simulink model "ADCS_Outline"  (R2019a)
settings: Solver=VariableStepAuto  StartTime=0.0  StopTime=duration  MaxStep=step
InitFcn:
  | SC_ODIN_INITIALIZATION
values from neighbouring files (symbols this model uses):
  A = [ v(1) v(4) v(5) v(7);        v(4) v(2) v(6) v(8);        v(5) v(6) v(3) v(9);        v(7) v(8) v(9) v(10) ]    [MagnetometerCalibration.m]    (also in SC_ODIN_INITIALIZATION.m = 0.06; test.m = asin(sin(N)/sin(n)*sin(a)))
  Amag = [0.910186583854  -0.00959593267728  0.00343590491018; -0.00959593267728  1.05471221352  0.0559849466324; 0.00343590491018  0.0559849466324  1.05528532305]    [MagnetometerBias.mat]    (also in MagnetometerCalibration.m = evecs/scale*evecs')
  argentina = [1612.36;-4182.16;-4522.83]    [SC_ODIN_INITIALIZATION.m]
  As = 0.2*0.3    (= 0.06)    [SC_ODIN_INITIALIZATION.m]
  b_mag = block.InputPort(3).Data    [MagnetometerCalibration.m]    (also in SC_ODIN_INITIALIZATION.m = [10;-15.5;-12.2]*1e-6)
  bmag = [1.00003671399e-05 -1.55007781395e-05 -1.22009762149e-05]    [MagnetometerBias.mat]    (also in MagnetometerCalibration.m = centerE)
  breakpoints = data(:,1)    [SC_ODIN_INITIALIZATION.m]
  c = 2.99792458e8    (= 299792458)    [SC_ODIN_INITIALIZATION.m]
  C_I = [0.045 0.0009 -0.00007;        0.0009 0.045 -0.00003;        -0.00007 -0.00003 0.009]    [SC_ODIN_INITIALIZATION.m]
  Cd = 2.0    (= 2)    [SC_ODIN_INITIALIZATION.m]
  controller_sample_rate = 0.5    [SC_ODIN_INITIALIZATION.m]
  D = [ 2 * x,            2 * y,            2 * z,            1 + 0 * x ]    [MagnetometerCalibration.m]    (also in SC_ODIN_INITIALIZATION.m = 0.01*[1;1;1])
  datapx = data(:,2)    [SC_ODIN_INITIALIZATION.m]
  datapy = data(:,3)    [SC_ODIN_INITIALIZATION.m]
  datapz = data(:,4)    [SC_ODIN_INITIALIZATION.m]
  datavx = data(:,5)    [SC_ODIN_INITIALIZATION.m]
  datavy = data(:,6)    [SC_ODIN_INITIALIZATION.m]
  datavz = data(:,7)    [SC_ODIN_INITIALIZATION.m]
  DCM_BT0 = eye(3)    [SC_ODIN_INITIALIZATION.m]
  G = 6.67408e-11    [SC_ODIN_INITIALIZATION.m]
  ground = [1266.06;-4295.81;4526.14]    [SC_ODIN_INITIALIZATION.m]
  I = [Ixx -Ixy -Ixz;      -Ixy Iyy -Iyz;      -Ixz -Iyz Izz]    [SC_ODIN_INITIALIZATION.m]
  invA_mag = block.InputPort(2).Data    [MagnetometerCalibration.m]    (also in SC_ODIN_INITIALIZATION.m = inv(Ellrot/scale*Ellrot'))
  JD_0 = start_day+start_fraction    [SC_ODIN_INITIALIZATION.m]
  Ks = 1367    [SC_ODIN_INITIALIZATION.m]
  L = [0.0000812 -0.0022136 -0.0225868]    [SC_ODIN_INITIALIZATION.m]
  Ls = 0.01*[-3; 3; 5]    [SC_ODIN_INITIALIZATION.m]
  M = 5.9722e24    (= 5.9722e+24)    [SC_ODIN_INITIALIZATION.m]    (also in visualisation.m = uicontrol('Style','text','String',{''},'Position',[710 100+2)
  magnetorquer_tau = 0.02    [SC_ODIN_INITIALIZATION.m]
  magnetorquer_x_saturation = 0.24    [SC_ODIN_INITIALIZATION.m]
  magnetorquer_y_saturation = 0.24    [SC_ODIN_INITIALIZATION.m]
  magnetorquer_z_saturation = 0.13    [SC_ODIN_INITIALIZATION.m]
  namibia = [5659.26;1238.85;-2659.2]    [SC_ODIN_INITIALIZATION.m]
  q = 0.6    [SC_ODIN_INITIALIZATION.m]
  radii = radii .* sgns    [MagnetometerCalibration.m]    (also in SC_ODIN_INITIALIZATION.m = [1;0.9;1.1])
  W0 = [1;0;1-1/240].*pi()/180    [SC_ODIN_INITIALIZATION.m]
  wheel_saturation = 0.23e-3    (= 0.00023)    [SC_ODIN_INITIALIZATION.m]
  wheel_tau = 2    [SC_ODIN_INITIALIZATION.m]
undefined symbols (not defined in the file or in its folder): DiscIntNeverNeededParam, nut80, sun_sensors
libraries: dspmathops x94, vrlib x70, dspsrcs4 x21, realtime_pacer_lib x1, dspsolvers x1, dspinverses x1
(part 3 of 6)

== system ADCS_Outline/Guidance&Determination/Body-Earth Estimation/TRIAD DCM ==
  (Sx,Sy,Sz) : Inport
  " (Bx,By,Bz)" : Inport  Port=2
  (Sxe,Sye,Sze) : Inport  Port=3
  (Bxe,Bye,Bze) : Inport  Port=4
  Cross Product{,1..3} (4 alike) : vrlib/Utilities/Cross Product
      settings: SourceProductBaseCode=VR
  Matrix Concatenate : Concatenate  NumInputs=3  Mode=Multidimensional array  ConcatenateDimension=2
  Matrix Concatenate1 : Concatenate  NumInputs=3  Mode=Multidimensional array  ConcatenateDimension=2
  Matrix Multiply : Product  Multiplication=Matrix(*)
  Normalization{,1..5} (6 alike) : dspmathops/Normalization  NormType=2-norm  Bias=1e-10  NormOver=Each column  Dimension=1  roundingMode=Floor  overflowMode=off  accumDataTypeStr=Inherit: Same as product output  accumLastDataTypeStr=Inherit: Same as product output  outputDataTypeStr=Inherit: Same as product output  outputMin=[]  outputMax=[]  outputLastDataTypeStr=Inherit: Same as product output
      settings: SourceProductName=DSP System Toolbox
  Signal Specification1 : SignalSpecification  Dimensions=3
  Transpose : Math  Operator=transpose  SaturateOnIntegerOverflow=on
  DCM BE : Outport
  wires:
  Normalization/1 -> Matrix Concatenate/3, Cross Product1/1
  Normalization5/1 -> Matrix Concatenate1/1, Cross Product3/2
  Cross Product1/1 -> Normalization1/1
  Normalization3/1 -> Matrix Concatenate1/2
  Cross Product3/1 -> Signal Specification1/1
  (Bxe,Bye,Bze)/1 -> Cross Product/2
  Normalization4/1 -> Matrix Concatenate/1, Cross Product1/2
  (Sxe,Sye,Sze)/1 -> Normalization4/1, Cross Product/1
  Cross Product2/1 -> Normalization2/1
  Cross Product/1 -> Normalization/1
  Normalization1/1 -> Matrix Concatenate/2
  Normalization2/1 -> Cross Product3/1, Matrix Concatenate1/3
  Matrix Concatenate/1 -> Transpose/1
  Matrix Concatenate1/1 -> Matrix Multiply/1
  Transpose/1 -> Matrix Multiply/2
  (Sx,Sy,Sz)/1 -> Cross Product2/1, Normalization5/1
  " (Bx,By,Bz)"/1 -> Cross Product2/2
  Matrix Multiply/1 -> DCM BE/1
  Signal Specification1/1 -> Normalization3/1

== system ADCS_Outline/Guidance&Determination/Guidance/TRIAD ==
  PointingE : Inport
  ConstraintE : Inport  Port=2
  PointingB : Inport  Port=3
  ContraintB : Inport  Port=4
  " " : MATLAB Function  TreatAsAtomicUnit=on
  Cross Product{,1..3} (4 alike) : vrlib/Utilities/Cross Product
      settings: SourceProductBaseCode=VR
  Matrix Concatenate : Concatenate  NumInputs=3  Mode=Multidimensional array  ConcatenateDimension=2
  Matrix Concatenate1 : Concatenate  NumInputs=3  Mode=Multidimensional array  ConcatenateDimension=2
  Matrix Multiply : Product  Multiplication=Matrix(*)
  Normalization{,1..5} (6 alike) : dspmathops/Normalization  NormType=2-norm  Bias=1e-10  NormOver=Each column  Dimension=1  roundingMode=Floor  overflowMode=off  accumDataTypeStr=Inherit: Same as product output  accumLastDataTypeStr=Inherit: Same as product output  outputDataTypeStr=Inherit: Same as product output  outputMin=[]  outputMax=[]  outputLastDataTypeStr=Inherit: Same as product output
      settings: SourceProductName=DSP System Toolbox
  Signal Specification1 : SignalSpecification  Dimensions=3
  Transpose : Math  Operator=transpose  SaturateOnIntegerOverflow=on
  q_ET : Outport
  wires:
  Signal Specification1/1 -> Normalization3/1
  ConstraintE/1 -> Cross Product2/2
  PointingE/1 -> Normalization5/1, Cross Product2/1
  Transpose/1 -> Matrix Multiply/2
  Matrix Concatenate1/1 -> Matrix Multiply/1
  Matrix Concatenate/1 -> Transpose/1
  Normalization2/1 -> Cross Product3/1, Matrix Concatenate1/3
  Normalization1/1 -> Matrix Concatenate/2
  Cross Product/1 -> Normalization/1
  Cross Product2/1 -> Normalization2/1
  PointingB/1 -> Cross Product/1, Normalization4/1
  Normalization4/1 -> Cross Product1/2, Matrix Concatenate/1
  ContraintB/1 -> Cross Product/2
  Cross Product3/1 -> Signal Specification1/1
  Normalization3/1 -> Matrix Concatenate1/2
  Cross Product1/1 -> Normalization1/1
  Normalization5/1 -> Cross Product3/2, Matrix Concatenate1/1
  Normalization/1 -> Cross Product1/1, Matrix Concatenate/3
  Matrix Multiply/1 -> " "/1(dcm)
  " "/1(q) -> q_ET/1

== system ADCS_Outline/Guidance&Determination/TargetFrameVelocity/Filtered Derivative1 ==
  x : Inport
  Add : Sum  Inputs=-+
  Discrete-Time Integrator : DiscreteIntegrator  SampleTime=-1  ICPrevOutput=DiscIntNeverNeededParam  ICPrevScaledInput=DiscIntNeverNeededParam
  Time Constant (1/tau) : Gain
  dx : Outport
  wires:
  Discrete-Time Integrator/1 -> Add/1
  Time Constant (1/tau)/1 -> Discrete-Time Integrator/1, dx/1
  Add/1 -> Time Constant (1/tau)/1
  x/1 -> Add/2

== system ADCS_Outline/Magnetometer /Calibration (Calculated onboard)/Calibration ==
  note: For comparison to real values
  C(Bx,By,Bz) : Inport
  Mode : Inport  Port=2
  B_E : Inport  Port=3
  Constant : Constant  Value=invA_mag
  Constant1 : Constant  Value=b_mag
  Constant2 : Constant  Value=radii
  Level-2 MATLAB S-Function : M-S-Function  FunctionName=MagnetometerCalibration  Parameters=""
  wires:
  C(Bx,By,Bz)/1 -> Level-2 MATLAB S-Function/1
  Constant/1 -> Level-2 MATLAB S-Function/2
  Constant1/1 -> Level-2 MATLAB S-Function/3
  Mode/1 -> Level-2 MATLAB S-Function/5
  Constant2/1 -> Level-2 MATLAB S-Function/4
  B_E/1 -> Level-2 MATLAB S-Function/6

== system ADCS_Outline/Momentum Control/Bdot Controller/Arduino ==
  C(Bx,By,Bz) : Inport  LatchByDelayingOutsideSignal=on
  Trigger : TriggerPort  VariantControl=Variant  PortDimensions=1
  Arduino : MATLABFcn  MATLABFcn=Bdot_Arduino
  C(Mx,My,Mz) : Outport
  wires:
  Arduino/1 -> C(Mx,My,Mz)/1
  C(Bx,By,Bz)/1 -> Arduino/1

== system ADCS_Outline/Momentum Control/Bdot Controller/Bang Bang Controller ==
  C(Bdotx,Bdoty,Bdotz) : Inport
  Dot Product : DotProduct  InputSameDT=on  OutDataTypeStr=Inherit: Inherit via internal rule
  Dot Product1 : DotProduct  InputSameDT=on  OutDataTypeStr=Inherit: Inherit via internal rule
  Dot Product2 : DotProduct  InputSameDT=on  OutDataTypeStr=Inherit: Inherit via internal rule
  Gain : Gain  Gain=magnetorquer_x_saturation
  Gain1 : Gain  Gain=magnetorquer_y_saturation
  Gain2 : Gain  Gain=magnetorquer_z_saturation
  Gain3 : Gain  Gain=-1
  Magnetoquer x : Constant  Value=[1,0,0]
  Magnetoquer x1 : Constant  Value=[0,1,0]
  Magnetoquer x2 : Constant  Value=[0,0,1]
  Mux : Mux  Inputs=3
  Sign : Signum  ZeroCross=off
  Sign1 : Signum  ZeroCross=off
  Sign2 : Signum  ZeroCross=off
  C(mx,My,Mz) : Outport
  wires:
  Magnetoquer x/1 -> Dot Product/1
  C(Bdotx,Bdoty,Bdotz)/1 -> Dot Product1/2, Dot Product2/2, Dot Product/2
  Dot Product/1 -> Sign/1
  Sign/1 -> Gain/1
  Mux/1 -> Gain3/1
  Gain/1 -> Mux/1
  Gain1/1 -> Mux/2
  Magnetoquer x1/1 -> Dot Product1/1
  Sign1/1 -> Gain1/1
  Dot Product1/1 -> Sign1/1
  Gain2/1 -> Mux/3
  Magnetoquer x2/1 -> Dot Product2/1
  Sign2/1 -> Gain2/1
  Dot Product2/1 -> Sign2/1
  Gain3/1 -> C(mx,My,Mz)/1

== system ADCS_Outline/Momentum Control/Bdot Controller/Bang Bang with direction ==
  note: Scales the vector to its max length but keeps the same direction
  C(Mx,My,Mz) : Inport
  Demux : Demux  Outputs=3
  Divide : Product  Inputs=*/
  Gain : Gain  Gain=-1
  Max : MinMax  Function=max  Inputs=3
  Saturation x : Fcn  Expr=abs(u)/magnetorquer_x_saturation
  Saturation y : Fcn  Expr=abs(u)/magnetorquer_y_saturation
  Saturation z : Fcn  Expr=abs(u)/magnetorquer_z_saturation
  sat_C(Mx,My,Mz) : Outport
  wires:
  Demux/3 -> Saturation z/1
  Demux/1 -> Saturation x/1
  Saturation x/1 -> Max/1
  C(Mx,My,Mz)/1 -> Demux/1, Divide/1
  Saturation y/1 -> Max/2
  Max/1 -> Divide/2
  Divide/1 -> Gain/1
  Demux/2 -> Saturation y/1
  Saturation z/1 -> Max/3
  Gain/1 -> sat_C(Mx,My,Mz)/1

== system ADCS_Outline/Momentum Control/Bdot Controller/Filtered Derivative ==
  x : Inport
  Add : Sum  Inputs=-+
  Discrete-Time Integrator : DiscreteIntegrator  SampleTime=-1  ICPrevOutput=DiscIntNeverNeededParam  ICPrevScaledInput=DiscIntNeverNeededParam
  Time Constant (1/tau) : Gain  Gain=0.5
  dx : Outport
  wires:
  Discrete-Time Integrator/1 -> Add/1
  Time Constant (1/tau)/1 -> Discrete-Time Integrator/1, dx/1
  Add/1 -> Time Constant (1/tau)/1
  x/1 -> Add/2

== system ADCS_Outline/Momentum Control/Bdot Controller/Saturation ==
  note: Trims the vector but keeps the same direction
  C(Mx,My,Mz) : Inport
  Demux : Demux  Outputs=3
  Divide : Product  Inputs=*/
  Max : MinMax  Function=max  Inputs=4
  Not saturated : Constant
  Saturation x : Fcn  Expr=abs(u)/magnetorquer_x_saturation
  Saturation y : Fcn  Expr=abs(u)/magnetorquer_y_saturation
  Saturation z : Fcn  Expr=abs(u)/magnetorquer_z_saturation
  sat_C(Mx,My,Mz) : Outport
  wires:
  Saturation z/1 -> Max/3
  Demux/2 -> Saturation y/1
  Max/1 -> Divide/2
  Saturation y/1 -> Max/2
  Saturation x/1 -> Max/1
  Demux/1 -> Saturation x/1
  Demux/3 -> Saturation z/1
  C(Mx,My,Mz)/1 -> Divide/1, Demux/1
  Divide/1 -> sat_C(Mx,My,Mz)/1
  Not saturated/1 -> Max/4

== system ADCS_Outline/Momentum Control/Momentum Bias/Rotation ==
  q : Inport
  vi : Inport  Port=2
  "    " : MATLAB Function  TreatAsAtomicUnit=on
  "    1" : MATLAB Function  TreatAsAtomicUnit=on
  Constant : Constant  Value=[-1 -1 -1 1]
  Demux : Demux
  MATLAB Function : MATLAB Function  TreatAsAtomicUnit=on
  Multiply : Product
  Mux : Mux  Inputs=3
  Signal Specification : SignalSpecification  Dimensions=[1 4]
  Terminator : Terminator
  vo : Outport
  wires:
  Constant/1 -> Multiply/1
  q/1 -> Multiply/2, "    "/1(qa)
  vi/1 -> MATLAB Function/1(u)
  "    "/1(q) -> Signal Specification/1
  Multiply/1 -> "    1"/2(qb)
  MATLAB Function/1(y) -> "    "/2(qb)
  Mux/1 -> vo/1
  "    1"/1(q) -> Demux/1
  Demux/1 -> Mux/1
  Demux/2 -> Mux/2
  Demux/3 -> Mux/3
  Demux/4 -> Terminator/1
  Signal Specification/1 -> "    1"/1(qa)

== system ADCS_Outline/Toolbox/DCM2W/Anti-Skewed ==
  note: This constant is useless but fixes an initial dimension issue with simulink
  m : Inport
  Add : Sum
  Constant : Constant  Value=zeros(3,3)
  MATLAB Function : MATLAB Function  TreatAsAtomicUnit=on
  v : Outport
  wires:
  MATLAB Function/1(y) -> v/1
  Add/1 -> MATLAB Function/1(u)
  m/1 -> Add/2
  Constant/1 -> Add/1

== system ADCS_Outline/Toolbox/DCM2W/Filtered Derivative ==
  x : Inport
  Add : Sum  Inputs=-+
  Gain : Gain  Gain=5
  Integrator : Integrator
  dx : Outport
  wires:
  Integrator/1 -> Add/1
  Gain/1 -> Integrator/1, dx/1
  Add/1 -> Gain/1
  x/1 -> Add/2

== system ADCS_Outline/Toolbox/EKF Test/Quat Rot ==
  q : Inport
  vi : Inport  Port=2
  "    " : MATLAB Function  TreatAsAtomicUnit=on
  "    1" : MATLAB Function  TreatAsAtomicUnit=on
  Constant : Constant  Value=[-1 -1 -1 1]
  Demux : Demux
  MATLAB Function : MATLAB Function  TreatAsAtomicUnit=on
  Multiply : Product
  Mux : Mux  Inputs=3
  Terminator : Terminator
  vo : Outport
  wires:
  Constant/1 -> Multiply/1
  q/1 -> Multiply/2, "    "/1(qa)
  vi/1 -> MATLAB Function/1(u)
  "    "/1(q) -> "    1"/1(qa)
  Multiply/1 -> "    1"/2(qb)
  MATLAB Function/1(y) -> "    "/2(qb)
  Mux/1 -> vo/1
  "    1"/1(q) -> Demux/1
  Demux/1 -> Mux/1
  Demux/2 -> Mux/2
  Demux/3 -> Mux/3
  Demux/4 -> Terminator/1

== system ADCS_Outline/Toolbox/EKF Test/Quat Rot1 ==
  q : Inport
  vi : Inport  Port=2
  "    " : MATLAB Function  TreatAsAtomicUnit=on
  "    1" : MATLAB Function  TreatAsAtomicUnit=on
  Constant : Constant  Value=[-1 -1 -1 1]
  Demux : Demux
  MATLAB Function : MATLAB Function  TreatAsAtomicUnit=on
  Multiply : Product
  Mux : Mux  Inputs=3
  Terminator : Terminator
  vo : Outport
  wires:
  Demux/4 -> Terminator/1
  Demux/3 -> Mux/3
  Demux/2 -> Mux/2
  Demux/1 -> Mux/1
  "    1"/1(q) -> Demux/1
  Mux/1 -> vo/1
  MATLAB Function/1(y) -> "    "/2(qb)
  Multiply/1 -> "    1"/2(qb)
  "    "/1(q) -> "    1"/1(qa)
  vi/1 -> MATLAB Function/1(u)
  q/1 -> "    "/1(qa), Multiply/2
  Constant/1 -> Multiply/1

== system ADCS_Outline/Toolbox/EKF Test/S//C Kinematics ==
  (wx,wy,wz) : Inport
  xhat : Inport  Port=2
  Add : Sum
  Gain : Gain  Gain=0.5
  Gain1 : Gain  Gain=controller_sample_rate
  Matrix Multiply : Product  Multiplication=Matrix(*)
  Skewed : Subsystem
  q_BT : Outport
  wires:
  (wx,wy,wz)/1 -> Skewed/1(v)
  xhat/1 -> Add/2, Gain/1
  Skewed/1(m) -> Matrix Multiply/1
  Gain/1 -> Matrix Multiply/2
  Matrix Multiply/1 -> Gain1/1
  Gain1/1 -> Add/1
  Add/1 -> q_BT/1

== system ADCS_Outline/Toolbox/EKF Test/SC Dynamics ==
  note: integrator
  note: integrator
  C(Twx,Twy,Twz)i : Inport
  (Lwx,Lwy,Lwz)i : Inport  Port=2
  (wx,wy,wz)i : Inport  Port=3
  Add : Sum  Inputs=--
  Add1 : Sum
  Add3 : Sum
  Add4 : Sum
  Cross Product : vrlib/Utilities/Cross Product
      settings: SourceProductBaseCode=VR
  Delay One Step : Delay  DelayLength=1
  Gain : Gain  Gain=controller_sample_rate
  Gain1 : Gain  Gain=controller_sample_rate
  Inertia matrix I : Constant  Value=C_I
  Inverse of I : Constant  Value=inv(C_I)
  Matrix Multiply : Product  Multiplication=Matrix(*)
  Matrix Multiply1 : Product  Multiplication=Matrix(*)
  (wx,wy,wz) : Outport
  C(Ltx,Lty,Ltz) : Outport  Port=2
  wires:
  Add/1 -> Gain/1  "I*w_dot"
  Cross Product/1 -> Add/2
  Add3/1 -> Add1/2, Matrix Multiply/2  "I*w SC L"
  Inverse of I/1 -> Matrix Multiply/1
  Inertia matrix I/1 -> Matrix Multiply1/1
  Matrix Multiply/1 -> (wx,wy,wz)/1  "w"
  Matrix Multiply1/1 -> Add3/2
  (wx,wy,wz)i/1 -> Matrix Multiply1/2, Cross Product/1
  C(Twx,Twy,Twz)i/1 -> Gain1/1, Add/1
  Add4/1 -> Add1/1  "I*wh Wheels Lw"
  Add1/1 -> C(Ltx,Lty,Ltz)/1, Delay One Step/1
  (Lwx,Lwy,Lwz)i/1 -> Add4/2
  Gain/1 -> Add3/1
  Gain1/1 -> Add4/1
  Delay One Step/1 -> Cross Product/2

== system ADCS_Outline/Toolbox/No Control fast STK attitude recoding/   DCM EF ==
  (Vxe,Xye,Vze) : Inport
  (Pxe,Pye,Pze) : Inport  Port=2
  Constant : Constant  Value=[1;0;0]
  Constant1 : Constant  Value=[0;0;1]
  Cross Product{,1..3} (4 alike) : vrlib/Utilities/Cross Product
      settings: SourceProductBaseCode=VR
  Matrix Concatenate : Concatenate  NumInputs=3  Mode=Multidimensional array  ConcatenateDimension=2
  Matrix Concatenate1 : Concatenate  NumInputs=3  Mode=Multidimensional array  ConcatenateDimension=2
  Matrix Multiply : Product  Multiplication=Matrix(*)
  Normalization{,1..5} (6 alike) : dspmathops/Normalization  NormType=2-norm  Bias=1e-10  NormOver=Each column  Dimension=1  roundingMode=Floor  overflowMode=off  accumDataTypeStr=Inherit: Same as product output  accumLastDataTypeStr=Inherit: Same as product output  outputDataTypeStr=Inherit: Same as product output  outputMin=[]  outputMax=[]  outputLastDataTypeStr=Inherit: Same as product output
      settings: SourceProductName=DSP System Toolbox
  Signal Specification1 : SignalSpecification  Dimensions=3
  Transpose : Math  Operator=transpose  SaturateOnIntegerOverflow=on
  DCM EF : Outport
  wires:
  Normalization/1 -> Matrix Concatenate/3, Cross Product1/1
  Normalization5/1 -> Matrix Concatenate1/1, Cross Product3/2
  Cross Product1/1 -> Normalization1/1
  Normalization3/1 -> Matrix Concatenate1/2
  Cross Product3/1 -> Signal Specification1/1
  Constant1/1 -> Cross Product/2
  Normalization4/1 -> Matrix Concatenate/1, Cross Product1/2
  Constant/1 -> Normalization4/1, Cross Product/1
  Cross Product2/1 -> Normalization2/1
  Cross Product/1 -> Normalization/1
  Normalization1/1 -> Matrix Concatenate/2
  Normalization2/1 -> Cross Product3/1, Matrix Concatenate1/3
  Matrix Concatenate/1 -> Transpose/1
  Matrix Concatenate1/1 -> Matrix Multiply/1
  Transpose/1 -> Matrix Multiply/2
  (Vxe,Xye,Vze)/1 -> Cross Product2/1, Normalization5/1
  (Pxe,Pye,Pze)/1 -> Cross Product2/2
  Matrix Multiply/1 -> DCM EF/1
  Signal Specification1/1 -> Normalization3/1

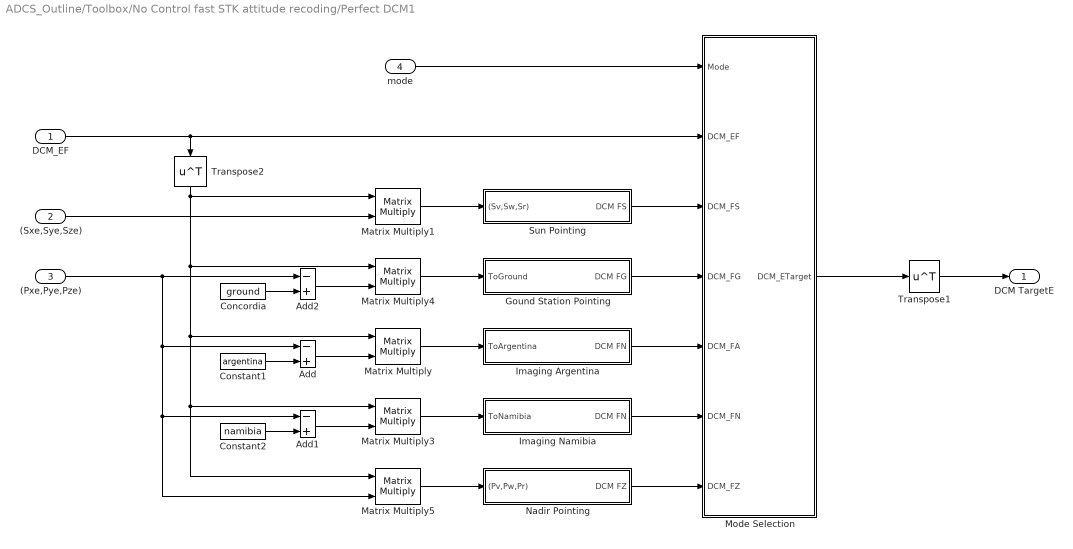
== system ADCS_Outline/Toolbox/No Control fast STK attitude recoding/Perfect DCM1 ==
  "DCM_EF " : Inport
  (Sxe,Sye,Sze) : Inport  Port=2
  (Pxe,Pye,Pze) : Inport  Port=3
  mode : Inport  Port=4
  " Imaging Argentina" : Subsystem
  " Imaging Namibia" : Subsystem
  " Nadir Pointing" : Subsystem
  Add : Sum  Inputs=-+
  Add1 : Sum  Inputs=-+
  Add2 : Sum  Inputs=-+
  Concordia : Constant  Value=ground
  Constant1 : Constant  Value=argentina
  Constant2 : Constant  Value=namibia
  Gound Station Pointing : Subsystem
  Matrix Multiply{,1,3..5} (5 alike) : Product  Multiplication=Matrix(*)
  Mode Selection : MATLAB Function  TreatAsAtomicUnit=on
  Sun Pointing : Subsystem
  Transpose1 : Math  Operator=transpose  SaturateOnIntegerOverflow=on
  Transpose2 : Math  Operator=transpose  SaturateOnIntegerOverflow=on
  DCM TargetE : Outport
  wires:
  mode/1 -> Mode Selection/1(Mode)
  Mode Selection/1(DCM_ETarget) -> Transpose1/1
  " Nadir Pointing"/1(DCM FZ) -> Mode Selection/7(DCM_FZ)
  " Imaging Namibia"/1(DCM FN) -> Mode Selection/6(DCM_FN)
  " Imaging Argentina"/1(DCM FN) -> Mode Selection/5(DCM_FA)
  Gound Station Pointing/1(DCM FG) -> Mode Selection/4(DCM_FG)
  Sun Pointing/1(DCM FS) -> Mode Selection/3(DCM_FS)
  (Sxe,Sye,Sze)/1 -> Matrix Multiply1/2
  Constant1/1 -> Add/2
  Concordia/1 -> Add2/2
  Matrix Multiply5/1 -> " Nadir Pointing"/1((Pv,Pw,Pr))
  Matrix Multiply4/1 -> Gound Station Pointing/1(ToGround)
  Add2/1 -> Matrix Multiply4/2
  Matrix Multiply3/1 -> " Imaging Namibia"/1(ToNamibia)
  (Pxe,Pye,Pze)/1 -> Matrix Multiply5/2, Add1/1, Add/1, Add2/1
  Matrix Multiply/1 -> " Imaging Argentina"/1(ToArgentina)
  Add/1 -> Matrix Multiply/2
  Constant2/1 -> Add1/2
  Add1/1 -> Matrix Multiply3/2
  Transpose1/1 -> DCM TargetE/1
  "DCM_EF "/1 -> Transpose2/1, Mode Selection/2(DCM_EF)
  Matrix Multiply1/1 -> Sun Pointing/1((Sv,Sw,Sr))
  Transpose2/1 -> Matrix Multiply1/1, Matrix Multiply5/1, Matrix Multiply3/1, Matrix Multiply/1, Matrix Multiply4/1

== system ADCS_Outline/Toolbox/No Control fast STK attitude recoding/STK Attitude Recording1 ==
  DCM_BE : Inport
  Mode : Inport  Port=2
  Clock : Clock
  DCM to q : MATLAB Function  TreatAsAtomicUnit=on
  MATLAB Function : MATLAB Function  TreatAsAtomicUnit=on
  Mux : Mux  Inputs=2
  Pulse Generator : DiscretePulseGenerator  PulseType=Time based  Period=180  PulseWidth=5  PhaseDelay=1e-16
  Pulse Generator1 : DiscretePulseGenerator  PulseType=Time based  PulseWidth=5  PhaseDelay=1e-16
  Subsystem : Subsystem
  Switch : Switch  Threshold=1
  wires:
  DCM to q/1(q) -> Mux/2
  Clock/1 -> Mux/1
  DCM_BE/1 -> DCM to q/1(dcm_inv)
  Mux/1 -> Subsystem/1(q_EB)
  Pulse Generator1/1 -> Switch/3
  Pulse Generator/1 -> Switch/1
  Mode/1 -> MATLAB Function/1(u)
  MATLAB Function/1(y) -> Switch/2
  Switch/1 -> Subsystem/Trigger

== system ADCS_Outline/Toolbox/S//C Kinematics1/Skewed ==
  v : Inport
  MATLAB Function : MATLAB Function  TreatAsAtomicUnit=on
  m : Outport
  wires:
  v/1 -> MATLAB Function/1(u)
  MATLAB Function/1(y) -> m/1

== system ADCS_Outline/Toolbox/S//C Kinematics2/Skewed ==
  v : Inport
  MATLAB Function : MATLAB Function  TreatAsAtomicUnit=on
  m : Outport
  wires:
  v/1 -> MATLAB Function/1(u)
  MATLAB Function/1(y) -> m/1

== system ADCS_Outline/Toolbox/EKF Test/S//C Kinematics/Skewed ==
  v : Inport
  MATLAB Function : MATLAB Function  TreatAsAtomicUnit=on
  m : Outport
  wires:
  v/1 -> MATLAB Function/1(u)
  MATLAB Function/1(y) -> m/1

== system ADCS_Outline/Toolbox/No Control fast STK attitude recoding/Perfect DCM1/ Imaging Argentina ==
  ToArgentina : Inport
  Constant : Constant  Value=[0;0;1]
  Constant1 : Constant  Value=[0;1;0]
  Cross Product{,1..3} (4 alike) : vrlib/Utilities/Cross Product
      settings: SourceProductBaseCode=VR
  Matrix Concatenate : Concatenate  NumInputs=3  Mode=Multidimensional array  ConcatenateDimension=2
  Matrix Concatenate1 : Concatenate  NumInputs=3  Mode=Multidimensional array  ConcatenateDimension=2
  Matrix Multiply : Product  Multiplication=Matrix(*)
  Normalization{,1..5} (6 alike) : dspmathops/Normalization  NormType=2-norm  Bias=1e-10  NormOver=Each column  Dimension=1  roundingMode=Floor  overflowMode=off  accumDataTypeStr=Inherit: Same as product output  accumLastDataTypeStr=Inherit: Same as product output  outputDataTypeStr=Inherit: Same as product output  outputMin=[]  outputMax=[]  outputLastDataTypeStr=Inherit: Same as product output
      settings: SourceProductName=DSP System Toolbox
  Signal Specification : SignalSpecification  Dimensions=3
  Signal Specification1 : SignalSpecification  Dimensions=3
  Transpose : Math  Operator=transpose  SaturateOnIntegerOverflow=on
  Velocity : Constant  Value=[1;0;0]
  DCM FN : Outport
  wires:
  Cross Product1/1 -> Normalization1/1
  Normalization5/1 -> Matrix Concatenate1/1, Cross Product3/2
  Normalization3/1 -> Matrix Concatenate1/2
  Velocity/1 -> Normalization5/1, Cross Product2/1
  Constant/1 -> Normalization4/1, Cross Product/1
  Normalization2/1 -> Cross Product3/1, Matrix Concatenate1/3
  Cross Product/1 -> Normalization/1
  Normalization1/1 -> Matrix Concatenate/2
  Cross Product2/1 -> Signal Specification/1
  Transpose/1 -> Matrix Multiply/2
  Normalization4/1 -> Matrix Concatenate/1, Cross Product1/2
  Matrix Concatenate/1 -> Transpose/1
  Matrix Concatenate1/1 -> Matrix Multiply/1
  Matrix Multiply/1 -> DCM FN/1
  Signal Specification/1 -> Normalization2/1
  Signal Specification1/1 -> Normalization3/1
  Normalization/1 -> Cross Product1/1, Matrix Concatenate/3
  ToArgentina/1 -> Cross Product2/2
  Cross Product3/1 -> Signal Specification1/1
  Constant1/1 -> Cross Product/2

== system ADCS_Outline/Toolbox/No Control fast STK attitude recoding/Perfect DCM1/ Imaging Namibia ==
  ToNamibia : Inport
  Constant : Constant  Value=[0;0;1]
  Constant1 : Constant  Value=[0;1;0]
  Cross Product{,1..3} (4 alike) : vrlib/Utilities/Cross Product
      settings: SourceProductBaseCode=VR
  Matrix Concatenate : Concatenate  NumInputs=3  Mode=Multidimensional array  ConcatenateDimension=2
  Matrix Concatenate1 : Concatenate  NumInputs=3  Mode=Multidimensional array  ConcatenateDimension=2
  Matrix Multiply : Product  Multiplication=Matrix(*)
  Normalization{,1..5} (6 alike) : dspmathops/Normalization  NormType=2-norm  Bias=1e-10  NormOver=Each column  Dimension=1  roundingMode=Floor  overflowMode=off  accumDataTypeStr=Inherit: Same as product output  accumLastDataTypeStr=Inherit: Same as product output  outputDataTypeStr=Inherit: Same as product output  outputMin=[]  outputMax=[]  outputLastDataTypeStr=Inherit: Same as product output
      settings: SourceProductName=DSP System Toolbox
  Signal Specification : SignalSpecification  Dimensions=3
  Signal Specification1 : SignalSpecification  Dimensions=3
  Transpose : Math  Operator=transpose  SaturateOnIntegerOverflow=on
  Velocity : Constant  Value=[1;0;0]
  DCM FN : Outport
  wires:
  Constant1/1 -> Cross Product/2
  Cross Product3/1 -> Signal Specification1/1
  ToNamibia/1 -> Cross Product2/2
  Normalization/1 -> Matrix Concatenate/3, Cross Product1/1
  Signal Specification1/1 -> Normalization3/1
  Signal Specification/1 -> Normalization2/1
  Matrix Multiply/1 -> DCM FN/1
  Matrix Concatenate1/1 -> Matrix Multiply/1
  Matrix Concatenate/1 -> Transpose/1
  Normalization4/1 -> Cross Product1/2, Matrix Concatenate/1
  Transpose/1 -> Matrix Multiply/2
  Cross Product2/1 -> Signal Specification/1
  Normalization1/1 -> Matrix Concatenate/2
  Cross Product/1 -> Normalization/1
  Normalization2/1 -> Matrix Concatenate1/3, Cross Product3/1
  Constant/1 -> Cross Product/1, Normalization4/1
  Velocity/1 -> Cross Product2/1, Normalization5/1
  Normalization3/1 -> Matrix Concatenate1/2
  Normalization5/1 -> Cross Product3/2, Matrix Concatenate1/1
  Cross Product1/1 -> Normalization1/1

== system ADCS_Outline/Toolbox/No Control fast STK attitude recoding/Perfect DCM1/ Nadir Pointing ==
  (Pv,Pw,Pr) : Inport
  Constant : Constant  Value=[0;0;1]
  Constant1 : Constant  Value=[0;-1;0]
  Cross Product{,1..3} (4 alike) : vrlib/Utilities/Cross Product
      settings: SourceProductBaseCode=VR
  Matrix Concatenate : Concatenate  NumInputs=3  Mode=Multidimensional array  ConcatenateDimension=2
  Matrix Concatenate1 : Concatenate  NumInputs=3  Mode=Multidimensional array  ConcatenateDimension=2
  Matrix Multiply : Product  Multiplication=Matrix(*)
  Normalization{,1..5} (6 alike) : dspmathops/Normalization  NormType=2-norm  Bias=1e-10  NormOver=Each column  Dimension=1  roundingMode=Floor  overflowMode=off  accumDataTypeStr=Inherit: Same as product output  accumLastDataTypeStr=Inherit: Same as product output  outputDataTypeStr=Inherit: Same as product output  outputMin=[]  outputMax=[]  outputLastDataTypeStr=Inherit: Same as product output
      settings: SourceProductName=DSP System Toolbox
  Signal Specification : SignalSpecification  Dimensions=3
  Signal Specification1 : SignalSpecification  Dimensions=3
  Transpose : Math  Operator=transpose  SaturateOnIntegerOverflow=on
  Velocity : Constant  Value=[1;0;0]
  DCM FZ : Outport
  wires:
  Cross Product1/1 -> Normalization1/1
  Normalization5/1 -> Matrix Concatenate1/1, Cross Product3/2
  Normalization3/1 -> Matrix Concatenate1/2
  Velocity/1 -> Normalization5/1, Cross Product2/1
  Constant/1 -> Normalization4/1, Cross Product/1
  Normalization2/1 -> Cross Product3/1, Matrix Concatenate1/3
  Cross Product/1 -> Normalization/1
  Normalization1/1 -> Matrix Concatenate/2
  Cross Product2/1 -> Signal Specification/1
  Transpose/1 -> Matrix Multiply/2
  Normalization4/1 -> Matrix Concatenate/1, Cross Product1/2
  Matrix Concatenate/1 -> Transpose/1
  Matrix Concatenate1/1 -> Matrix Multiply/1
  Matrix Multiply/1 -> DCM FZ/1
  Signal Specification/1 -> Normalization2/1
  Signal Specification1/1 -> Normalization3/1
  Normalization/1 -> Cross Product1/1, Matrix Concatenate/3
  (Pv,Pw,Pr)/1 -> Cross Product2/2
  Cross Product3/1 -> Signal Specification1/1
  Constant1/1 -> Cross Product/2

== system ADCS_Outline/Toolbox/No Control fast STK attitude recoding/Perfect DCM1/Gound Station Pointing ==
  ToGround : Inport
  Constant : Constant  Value=[0;1;0]
  Constant1 : Constant  Value=[0;0;1]
  Constant2 : Constant  Value=[1;0;0]
  Cross Product{,1..3} (4 alike) : vrlib/Utilities/Cross Product
      settings: SourceProductBaseCode=VR
  Matrix Concatenate : Concatenate  NumInputs=3  Mode=Multidimensional array  ConcatenateDimension=2
  Matrix Concatenate1 : Concatenate  NumInputs=3  Mode=Multidimensional array  ConcatenateDimension=2
  Matrix Multiply : Product  Multiplication=Matrix(*)
  Normalization{,1..5} (6 alike) : dspmathops/Normalization  NormType=2-norm  Bias=1e-10  NormOver=Each column  Dimension=1  roundingMode=Floor  overflowMode=off  accumDataTypeStr=Inherit: Same as product output  accumLastDataTypeStr=Inherit: Same as product output  outputDataTypeStr=Inherit: Same as product output  outputMin=[]  outputMax=[]  outputLastDataTypeStr=Inherit: Same as product output
      settings: SourceProductName=DSP System Toolbox
  Signal Specification : SignalSpecification  Dimensions=3
  Signal Specification1 : SignalSpecification  Dimensions=3
  Transpose : Math  Operator=transpose  SaturateOnIntegerOverflow=on
  DCM FG : Outport
  wires:
  Constant1/1 -> Cross Product/2
  Cross Product3/1 -> Signal Specification1/1
  Constant2/1 -> Cross Product2/2
  Normalization/1 -> Matrix Concatenate/3, Cross Product1/1
  Signal Specification1/1 -> Normalization3/1
  Signal Specification/1 -> Normalization2/1
  Matrix Multiply/1 -> DCM FG/1
  Matrix Concatenate1/1 -> Matrix Multiply/1
  Matrix Concatenate/1 -> Transpose/1
  Normalization4/1 -> Cross Product1/2, Matrix Concatenate/1
  Transpose/1 -> Matrix Multiply/2
  Cross Product2/1 -> Signal Specification/1
  Normalization1/1 -> Matrix Concatenate/2
  Cross Product/1 -> Normalization/1
  Normalization2/1 -> Matrix Concatenate1/3, Cross Product3/1
  Constant/1 -> Cross Product/1, Normalization4/1
  ToGround/1 -> Cross Product2/1, Normalization5/1
  Normalization3/1 -> Matrix Concatenate1/2
  Normalization5/1 -> Cross Product3/2, Matrix Concatenate1/1
  Cross Product1/1 -> Normalization1/1

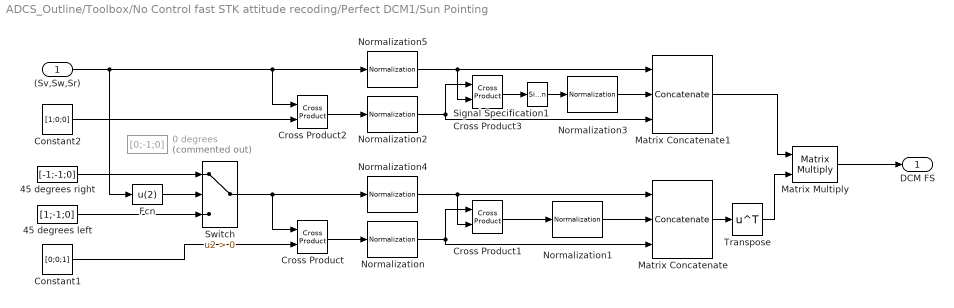
== system ADCS_Outline/Toolbox/No Control fast STK attitude recoding/Perfect DCM1/Sun Pointing ==
  (Sv,Sw,Sr) : Inport
  0 degrees : Constant  Commented=on  Value=[0;-1;0]
  45 degrees left : Constant  Value=[1;-1;0]
  45 degrees right : Constant  Value=[-1;-1;0]
  Constant1 : Constant  Value=[0;0;1]
  Constant2 : Constant  Value=[1;0;0]
  Cross Product{,1..3} (4 alike) : vrlib/Utilities/Cross Product
      settings: SourceProductBaseCode=VR
  Fcn : Fcn  Expr=u(2)
  Matrix Concatenate : Concatenate  NumInputs=3  Mode=Multidimensional array  ConcatenateDimension=2
  Matrix Concatenate1 : Concatenate  NumInputs=3  Mode=Multidimensional array  ConcatenateDimension=2
  Matrix Multiply : Product  Multiplication=Matrix(*)
  Normalization{,1..5} (6 alike) : dspmathops/Normalization  NormType=2-norm  Bias=1e-10  NormOver=Each column  Dimension=1  roundingMode=Floor  overflowMode=off  accumDataTypeStr=Inherit: Same as product output  accumLastDataTypeStr=Inherit: Same as product output  outputDataTypeStr=Inherit: Same as product output  outputMin=[]  outputMax=[]  outputLastDataTypeStr=Inherit: Same as product output
      settings: SourceProductName=DSP System Toolbox
  Signal Specification1 : SignalSpecification  Dimensions=3
  Switch : Switch  Criteria=u2 > Threshold
  Transpose : Math  Operator=transpose  SaturateOnIntegerOverflow=on
  DCM FS : Outport
  wires:
  Fcn/1 -> Switch/2
  45 degrees right/1 -> Switch/1
  45 degrees left/1 -> Switch/3
  Matrix Multiply/1 -> DCM FS/1
  Signal Specification1/1 -> Normalization3/1
  Constant2/1 -> Cross Product2/2
  (Sv,Sw,Sr)/1 -> Normalization5/1, Cross Product2/1, Fcn/1
  Transpose/1 -> Matrix Multiply/2
  Matrix Concatenate1/1 -> Matrix Multiply/1
  Matrix Concatenate/1 -> Transpose/1
  Normalization2/1 -> Matrix Concatenate1/3, Cross Product3/1
  Normalization1/1 -> Matrix Concatenate/2
  Cross Product/1 -> Normalization/1
  Cross Product2/1 -> Normalization2/1
  Switch/1 -> Cross Product/1, Normalization4/1
  Normalization4/1 -> Cross Product1/2, Matrix Concatenate/1
  Constant1/1 -> Cross Product/2
  Cross Product3/1 -> Signal Specification1/1
  Normalization3/1 -> Matrix Concatenate1/2
  Cross Product1/1 -> Normalization1/1
  Normalization5/1 -> Cross Product3/2, Matrix Concatenate1/1
  Normalization/1 -> Cross Product1/1, Matrix Concatenate/3

== system ADCS_Outline/Toolbox/No Control fast STK attitude recoding/STK Attitude Recording1/Subsystem ==
  q_EB : Inport
  Trigger : TriggerPort  VariantControl=Variant  PortDimensions=1
  To Workspace : ToWorkspace  VariableName=q_EB  SampleTime=-1
  wires:
  q_EB/1 -> To Workspace/1

== matlab function ADCS_Outline/Sun/MATLAB Function ==
  data: jd input; rsun output
%�
% ------------------------------------------------------------------------------
%
%                           function sunalmanac
%
%  this function calculates the geocentric equatorial position vector
%    the sun given the julian date.  this is the low precision formula and
%    is valid for years from 1950 to 2050.  accuaracy of apparent coordinates
%    is 0.01  degrees.  notice many of the calculations are performed in
%    degrees, and are not changed until later.  this is due to the fact that
%    the almanac uses degrees exclusively in their formulations.
%
%  author        : david vallado                  719-573-2600   27 may 2002
%
%  revisions
%    vallado     - fix mean lon of sun                            7 mat 2004
%
%  inputs          description                    range / units
%    jd          - julian date                    days from 4713 bc
%
%  outputs       :
%    rsun        - ijk position vector of the sun au
%    rtasc       - right ascension                rad
%    decl        - declination                    rad
%
%  locals        :
%    meanlong    - mean longitude
%    meananomaly - mean anomaly
%    eclplong    - ecliptic longitude
%    obliquity   - mean obliquity of the ecliptic
%    tut1        - julian centuries of ut1 from
%                  jan 1, 2000 12h
%    ttdb        - julian centuries of tdb from
%                  jan 1, 2000 12h
%    hr          - hours                          0 .. 24              10
%    min         - minutes                        0 .. 59              15
%    sec         - seconds                        0.0  .. 59.99          30.00
%    temp        - temporary variable
%    deg         - degrees
%
%  coupling      :
%    none.
%
%  references    :
%    vallado       2007, 281, alg 29, ex 5-1
%
% [rsun,rtasc,decl] = sunalmanac ( jd );
% ------------------------------------------------------------------------------

function rsun  = sunalmanac ( jd )

        twopi      =     2.0*pi;
        deg2rad    =     pi/180.0;

        % -------------------------  implementation   -----------------
        % -------------------  initialize values   --------------------
        tut1= ( jd - 2451545.0  )/ 36525.0;
% fprintf(1,'tut1 %14.9f \n',tut1);

        meanlong= 280.460  + 36000.771285*tut1;
        meanlong= rem( meanlong,360.0  );  %deg

        ttdb= tut1;
        meananomaly= 357.528  + 35999.050957 *ttdb;
        meananomaly= rem( meananomaly*deg2rad,twopi );  %rad
        if ( meananomaly < 0.0  )
            meananomaly= twopi + meananomaly;
        end

        eclplong= meanlong + 1.915 *sin(meananomaly) ...
                    + 0.020 *sin(2.0 *meananomaly); %deg
        eclplong= rem( eclplong,360.0  );  %deg

        obliquity= 23.439 - 0.01461 *ttdb;  %deg

        eclplong = eclplong *deg2rad;
        obliquity= obliquity *deg2rad;

        % --------- find magnitude of sun vector, )   components ------
        magr= 1.00014  - 0.01671 *cos( meananomaly ) ...
                              - 0.00014 *cos( 2.0 *meananomaly );    % in au's
        rsun = zeros(3,1);
        rsun(1,1)= magr*cos( eclplong );
        rsun(2,1)= magr*cos(obliquity)*sin(eclplong);
        rsun(3,1)= magr*sin(obliquity)*sin(eclplong);

% fprintf(1,'meanlon %11.6f meanan %11.6f eclplon %11.6f obli %11.6f \n', ...
%            meanlong,meananomaly/deg2rad,eclplong/deg2rad,obliquity/deg2rad);
% fprintf(1,'rs %11.9f %11.9f %11.9f \n',rsun);
% fprintf(1,'magr %14.7f \n',magr);

        rtasc= atan( cos(obliquity)*tan(eclplong) );

        % --- check that rtasc is in the same quadrant as eclplong ----
        if ( eclplong < 0.0  )
            eclplong= eclplong + twopi;    % make sure it's in 0 to 2pi range
        end
        if ( abs( eclplong-rtasc ) > pi*0.5  )
            rtasc= rtasc + 0.5 *pi*round( (eclplong-rtasc)/(0.5 *pi));
        end
        decl = asin( sin(obliquity)*sin(eclplong) );

== matlab function ADCS_Outline/DISTURBANCE TORQUES/ATMOSPHERIC DRAG/MATLAB Function ==
  data: h input; rho output
function rho = fcn(h)

%Reference altitude (km)

h_ref =linspace(250,500,11);

%Reference density (kg/m3)

rho_ref = [7.3e-11 4.1e-11 2.3e-11 1.38e-11 8.33e-12 5.24e-12,...
           3.29e-12 2.34e-12 1.39e-12 1e-12 6.15e-13];

%Interpolate based on altitude to find density   
       
rho = interp1(h_ref, rho_ref, h);

== matlab function ADCS_Outline/IGRF/MATLAB Function ==
  data: Bn output; latitude input; longitude input; altitude input; Be output; Bd output
function [Bn, Be, Bd] = igrf(latitude, longitude, altitude)

%REMOVED COORD AS EVERYTHING IS ALREADY IN GEOCENTRIC. KEEPING TIME FOR NOW

% IGRF Earth's magnetic field from IGRF model.
% 
% Usage: [BX, BY, BZ] = IGRF(TIME, LATITUDE, LONGITUDE, ALTITUDE, COORD)
%     or [BX, BY, BZ] = IGRF(COEFS, LATITUDE, LONGITUDE, ALTITUDE, COORD)
%     or B = IGRF(TIME, LATITUDE, LONGITUDE, ALTITUDE, COORD)
%     or B = IGRF(COEFS, LATITUDE, LONGITUDE, ALTITUDE, COORD)
% 
% Calculates the components of the Earth's magnetic field using the
% International Geomagnetic Reference Field (IGRF) model. The inputs for
% the position can be scalars or vectors (in the latter case each should
% have the same number of elements or be a scalar), but TIME must be a
% scalar.
% 
% When all the coordinate inputs are scalars, the function can be run more
% efficiently by providing the proper IGRF coefficient vector for a given
% time rather than the time itself. This mode is useful when making
% multiple calls to the function while keeping the time the same (meaning
% the coefficients will be the same for each run) as loading the
% coefficients can be the most time-consuming part of the function. The
% coefficient vector can be easily loaded using the function LOADIGRFCOEFS.
% This mode is assumed when all the coordinate inputs are scalars and the
% first input is a vector. In this case, the coefficient vector should be
% formatted as (LOADIGRFCOEFS provides this):
% 
%   [g(n=1,m=0) g(n=1,m=1) h(n=1,m=1) g(n=2,m=0) g(n=2,m=1) h(n=2,m=1) ...]
% 
% Regardless of the size of the inputs, the outputs will be column vectors.
% If only one output is requested, B = [BX(:), BY(:), BZ(:)] is output.
% Note that the other parameters the IGRF gives can be computed from BX,
% BY, and BZ as:
% 
%   Horizonal intensity: hypot(BX, BY) (i.e., sqrt(BX.^2 + BY.^2) )
%   Total intensity: hypot(BX, hypot(BY, BZ))
%   Declination: atan2(BY, BX)
%   Inclination: atan(BZ./hypot(BX, BY))
% 
% This function relies on having the file igrfcoefs.mat in the MATLAB
% path to function properly when a time is input. If this file cannot be
% found, this function will try to create it by calling GETIGRFCOEFS.
% 
% The IGRF is a spherical harmonic expansion of the Earth's internal
% magnetic field. Currently, the IGRF model is valid between the years 1900
% and 2015. See the health warning for the IGRF model here:
% http://www.ngdc.noaa.gov/IAGA/vmod/igrfhw.html
% 
% Reference:
% International Association of Geomagnetism and Aeronomy, Working Group 
% V-MOD (2010), International Geomagnetic Reference Field: the eleventh
% generation, _Geophys. J. Int._, _183_(3), 1216-1230, 
% doi:10.1111/j.1365-246X.2010.04804.x.
% 
% Inputs:
%   -TIME: Time to get the magnetic field values either in MATLAB serial
%   date number format or a string that can be converted into MATLAB serial
%   date number format using DATENUM with no format specified (see
%   documentation of DATENUM for more information).
%   -COEFS: Instead of inputting a time, you can simply specify the proper
%   coefficients for the time you want by inputting in the first argument
%   the proper coefficient vector from igrfcoefs.mat.
%   -LATITUDE: Geocentric or geodetic latitude in degrees. **SCODIN**In radian
%   -LONGITUDE: Geocentric or geodetic longitude in degrees. **SCODIN**In radian
%   -ALTITUDE: For geodetic coordiates, the height in km above the Earth's
%   surface. For geocentric coordiates, the radius in km from the center of
%   the Earth.
%   -COORD: String specifying the coordinate system to use. Either
%   'geocentric' or 'geodetic' (optional, default is geodetic). Note that
%   only geodetic coordinates have been verified.
% 
% Outputs:
%   -BX: Northward component of the magnetic field in nanoteslas (nT).
%   -BY: Eastward component of the magnetic field in nT.
%   -BZ: Downward component of the magnetic field in nT.
%   -B: [BX(:), BY(:), BZ(:)].
% 
% See also: LOADIGRFCOEFS, GETIGRFCOEFS, IGRFLINE, DATENUM, IGRF11MAGM.

% Run IGRFS if all position inputs are scalars.
if isscalar(latitude) && isscalar(longitude) && isscalar(altitude)
        [Bn, Be, Bd] = igrfs(latitude, longitude, altitude);
end

if nargout <= 1
    Bn = [Bn(:), Be(:), Bd(:)];
end
%%%%%%%%%%%%%%%%%%%%%%%%%%%%%%%%%%%%%%%%%%%%%%%%%%%%%%%%%%%%%%%%%%%%%%%%%%%
%%%%%%%%%%%%%%%%%%%        IGRF scalar function.        %%%%%%%%%%%%%%%%%%%
%%%%%%%%%%%%%%%%%%%%%%%%%%%%%%%%%%%%%%%%%%%%%%%%%%%%%%%%%%%%%%%%%%%%%%%%%%%
function [Bn, Be, Bd] = igrfs(latitude, longitude, altitude)

% Fundamental constant.
Rearth_km = 6371.2;

%%% CHECK INPUT VALIDITY %%%
% Convert time to a datenumber if it is a string.
% if ischar(time)
%     time = datenum(time);
% end

% Check that the input coordinates are scalars.
if ~isscalar(latitude) || ~isscalar(longitude) || ~isscalar(altitude)
    error('igrf1:inputNotScalar', ...
        'The input coordinates must be scalars.');
end

%%% SPHERICAL COORDINATE CONVERSION %%%
% Convert the latitude, longitude, and altitude coordinates input into
% spherical coordinates r (radius), theta (inclination angle from +z axis),
% and phi (azimuth angle from +x axis).
% We want cos(theta) and sin(theta) rather than theta itself.
costheta = cos(((pi()/2) - latitude));
sintheta = sin(((pi()/2) - latitude));

% Convert from geodetic coordinates to geocentric coordinates if necessary.
% This method was adapted from igrf11syn, which was a conversion of the
% IGRF subroutine written in FORTRAN.

r = altitude;

% Convert longitude to radians.
phi = longitude; %Conversion in Simulink

%IGRF Coefficient

gh = [-29442	-1501	4797.1	-2445.1	3012.9	-2845.6	1676.7	-641.9	1350.7	-2352.3	-115.3	1225.6	244.9	582	-538.4	907.6	813.7	283.3	120.4	-188.7	-334.9	180.9	70.4	-329.5	-232.6	360.1	47.3	192.4	197	-140.9	-119.3	-157.5	16	4.1	100.2	70	67.7	-20.8	72.7	33.2	-129.9	58.9	-28.9	-66.7	13.2	7.3	-70.9	62.6	81.6	-76.1	-54.1	-6.8	-19.5	51.8	5.7	15	24.4	9.4	3.4	-2.8	-27.4	6.8	-2.2	24.2	8.8	10.1	-16.9	-18.3	-3.2	13.3	-20.6	-14.6	13.4	16.2	11.7	5.7	-15.9	-9.1	-2	2.1	5.4	8.8	-21.6	3.1	10.8	-3.3	11.8	0.7	-6.8	-13.3	-6.9	-0.1	7.8	8.7	1	-9.1	-4	-10.5	8.4	-1.9	-6.3	3.2	0.1	-0.4	0.5	4.6	-0.5	4.4	1.8	-7.9	-0.7	-0.6	2.1	-4.2	2.4	-2.8	-1.8	-1.2	-3.6	-8.7	3.1	-1.5	-0.1	-2.3	2	2	-0.7	-0.8	-1.1	0.6	0.8	-0.7	-0.2	0.2	-2.2	1.7	-1.4	-0.2	-2.5	0.4	-2	3.5	-2.4	-1.9	-0.2	-1.1	0.4	0.4	1.2	1.9	-0.8	-2.2	0.9	0.3	0.1	0.7	0.5	-0.1	-0.3	0.3	-0.4	0.2	0.2	-0.9	-0.9	-0.1	0	0.7	0	-0.9	-0.9	0.4	0.4	0.5	1.6	-0.5	-0.5	1	-1.2	-0.2	-0.1	0.8	0.4	-0.1	-0.1	0.3	0.4	0.1	0.5	0.5	-0.3	-0.4	-0.4	-0.3	-0.8];
gh = transpose(gh);
nmax = sqrt(numel(gh) + 1) - 1;
% We need cos(m*phi) and sin(m*phi) multiple times, so precalculate into a
% vector here:
cosphi = cos((1:nmax)*phi);
sinphi = sin((1:nmax)*phi);

Pmax = (nmax+1)*(nmax+2)/2;

%%% BEGIN MAGNETIC FIELD CALCULATION %%%
% Initialize variables used in for loop below.
Br = 0; Bt = 0; Bp = 0;
 P = zeros(1, Pmax);  P(1) = 1;  P(3) = sintheta;
dP = zeros(1, Pmax); dP(1) = 0; dP(3) = costheta;

% For this initial condition, the first if will result in n = 1, m = 0.
m = 1; n = 0; coefindex = 1;

a_r = (Rearth_km/r)^2;

% Increment through all the n's and m's. gh will be a vector with g
% followed by h for incrementing through n and m except when h would be
% redundant (i.e., when m = 0).
for Pindex = 2:Pmax
    
    % Increment to the next n when m becomes larger than n.
    if n < m
        m = 0;
        n = n + 1;
        a_r = a_r*(Rearth_km/r); % We need (Rearth_km./r)^(n+2)
    end
    
    % Calculate P and dP. They are given recursively according to:
    % 
    % P(0, 0) = 1, P(1, 1) = sin(theta) <- Specified above
    % P(n, n) = sqrt(1 - 1/(2n))*sin(theta)*P(n-1, n-1)
    % P(n, m) = (2n - 1)/sqrt(n^2 - m^2)*cos(theta)*P(n-1, m) -
    %     sqrt(((n-1)^2 - m^2) / (n^2 - m^2)) * P(n-2, m)
    % 
    % dP(0, 0) = 0, dP(1, 1) = cos(theta) <- Specified above
    % dP(n, n) = sqrt(1 - 1/(2n))*(sin(theta)*dP(n-1, n-1) +
    %     cos(theta)*P(n-1, n-1))
    % dP(n, m) = (2n - 1)/sqrt(n^2 - m^2)*(cos(theta)*dP(n-1, m) -
    %     sin(theta)*P(n-1, m)) - sqrt(((n-1)^2 - m^2)/(n^2 - m^2))*
    %     dP(n-2, m)
    if m < n && Pindex ~= 3 % (Pindex=3 is n=1, m=1, initial cond. above)
        last1n = Pindex - n;
        last2n = Pindex - 2*n + 1;
        P(Pindex) = (2*n - 1)/sqrt(n^2 - m^2)*costheta*P(last1n) - ...
            sqrt(((n-1)^2 - m^2) / (n^2 - m^2)) * P(last2n);
        dP(Pindex) = (2*n - 1)/sqrt(n^2 - m^2)*(costheta*dP(last1n) - ...
            sintheta*P(last1n)) - sqrt(((n-1)^2 - m^2) / (n^2 - m^2)) * ...
            dP(last2n);
    elseif Pindex ~= 3
        lastn = Pindex - n - 1;
        P(Pindex) = sqrt(1 - 1/(2*m))*sintheta*P(lastn);
        dP(Pindex) = sqrt(1 - 1/(2*m))*(sintheta*dP(lastn) + ...
            costheta*P(lastn));
    end
    
    % Calculate the magnetic field components as a running sum. Find
    % explicit expressions for these in Global Earth Physics: a Handbook of
    % Physical Constants by Thomas J. Aherns (1995), pg. 49. Link:
    % http://books.google.com/books?id=aqjU_NHyre4C&lpg=PP1&dq=Global%20
    % earth%20physics%3A%20a%20handbook%20of%20physical%20constants&pg=PA49
    % #v=onepage&q&f=false
    % (except equation 6 is missing a required 1/sin(theta) and m; correct
    % equations on page 5 (equations 3a-3c) of:
    % http://hanspeterschaub.info/Papers/UnderGradStudents/
    % MagneticField.pdf)
    if m == 0 % Implies h = 0, so only coefficient in gh is g
        coef = a_r*gh(coefindex); %*cos(0*phi) = 1
        Br = Br + (n+1)*coef*P(Pindex);
        Bt = Bt - coef*dP(Pindex);
        % Bp is 0 for m = 0.
        coefindex = coefindex + 1; % Only need to skip over g this time.
    else
        coef = a_r*(gh(coefindex)*cosphi(m) + gh(coefindex+1)*sinphi(m));
        Br = Br + (n+1)*coef*P(Pindex);
        Bt = Bt - coef*dP(Pindex);
        if sintheta == 0 % Use different formula when dividing by 0.
            Bp = Bp - costheta*a_r*(-gh(coefindex)*sinphi(m) + ...
                gh(coefindex+1)*cosphi(m))*dP(Pindex);
        else
            Bp = Bp - 1/sintheta*a_r*m*(-gh(coefindex)*sinphi(m) + ...
                gh(coefindex+1)*cosphi(m))*P(Pindex);
        end
        coefindex = coefindex + 2; % Skip over g and h this time.
    end
    
    % Increment m.
    m = m + 1;
    
end

% Convert from spherical to (x,y,z) = (North,East,Down).
Bn = -Bt;
Be = Bp;
Bd = -Br;
